simulink model "IIR"  (R2020a)
settings: Solver=ode45  StartTime=0.0  StopTime=10000  RelTol=1e-3  EnableMultiTasking=on
PreLoadFcn:
  | IIR_PreLoadFcn
undefined symbols (not defined in the file): num_channels
libraries: xbsIndex_r4 x125, xbsCopyrightNotice_r4 x1
settings Model: Creator=alexc  LastModifiedBy=viswanad
settings DataIOCC: LimitDataPoints=on  SaveFormat=Array  SignalLoggingSaveFormat=ModelDataLogs  ReturnWorkspaceOutputs=off  SignalLoggingName=sigsOut
settings OptimizationCC: BlockReduction=off  BooleanDataType=off  DefaultParameterBehavior=Inlined  ExpressionDepthLimit=2147483647  InitFltsAndDblsToZero=on  LifeSpan=inf
settings DebuggingCC: SaveWithParameterizedLinksMsg=none  UnderspecifiedInitializationDetection=Classic  MergeDetectMultiDrivingBlocksExec=none  SignalResolutionControl=TryResolveAllWithWarning  MultiTaskDSMMsg=warning  MultiTaskCondExecSysMsg=none  FcnCallInpInsideContextMsg=warning  AllowSymbolicDim=off  StateNameClashWarn=warning  SFUnexpectedBacktrackingDiag=warning  SFNoUnconditionalDefaultTransitionDiag=warning  SFExecutionAtInitializationDiag=none  ArithmeticOperatorsInVariantConditions=warning
settings HardwareCC: ProdBitPerPointer=32  ProdBitPerSizeT=32  ProdBitPerPtrDiffT=32  ProdLargestAtomicFloat=None  ProdIntDivRoundTo=Undefined  ProdEndianess=Unspecified  ProdWordSize=32  ProdHWDeviceType=32-bit Generic  TargetUnknown=on
settings ModelReferenceCC: PropagateSignalLabelsOutOfModel=off
settings SFSimCC: SimUseLocalCustomCode=off  CustomCodeUndefinedFunction=UseInterfaceOnly
settings RTWCC: Description=Generic Real-Time Target  RTWUseLocalCustomCode=off
settings CodeAppCC: StateflowObjectComments=on
settings GRTTargetCC: TargetFcnLib=ansi_tfl_tmw.mat  TargetLangStandard=C89/C90 (ANSI)  CombineOutputUpdateFcns=off  GRTInterface=on
settings ConfigComp: CovMetricSettings=dw  CovSaveCumulativeToWorkspaceVar=on  CovSaveSingleToWorkspaceVar=on  CovExternalEMLEnable=off

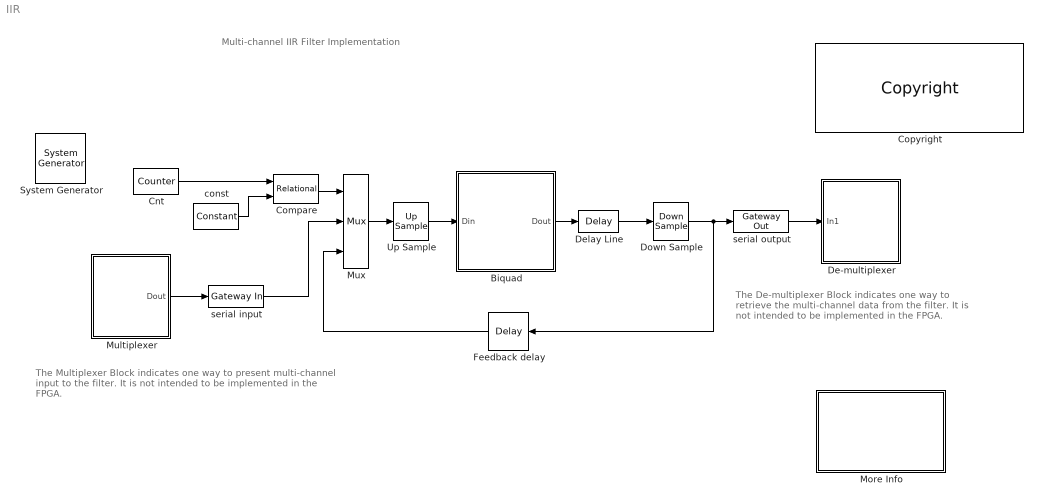
== system IIR ==
  note: Multi-channel IIR Filter Implementation
  note: The Multiplexer Block indicates one way to present
      | multi-channel input to the filter.  It is not intended to
      | be implemented in the FPGA.
  note: The De-multiplexer Block indicates one
      | way to retrieve the multi-channel data
      | from the filter. It is not intended to be
      | implemented in the FPGA.
  " System Generator" : xbsIndex_r4/ System Generator  Tag=genX  xilinxfamily=kintex7  part=xc7k325t  speed=-3  package=fbg676  synthesis_tool=Vivado  clock_wrapper=Clock Enables  directory=./netlist  proj_type=Vivado  Synth_file=Vivado Synthesis Defaults  Impl_file=Vivado Implementation Defaults  testbench=off  simulink_period=1  sysclk_period=22  dcm_input_clock_period=10  incr_netlist=off  trim_vbits=Everywhere in SubSystem  dbl_ovrd=According to Block Masks  core_generation=According to Block Masks  run_coregen=off  deprecated_control=off  eval_field=0  block_type=sysgen
  Biquad : Subsystem
  Cnt : xbsIndex_r4/Counter  cnt_type=Count Limited  cnt_to=4*num_channels-1  operation=Up  start_count=0  cnt_by_val=1  arith_type=Unsigned  n_bits=ceil(log2(4*num_channels))  bin_pt=0  load_pin=off  rst=off  en=off  explicit_period=on  period=5  use_behavioral_HDL=off  implementation=Fabric  use_rpm=off  XmcBlockStatus=1  maskContainerNames=group1  block_type=counter  block_config=sysgen:Counter_config
  Compare : xbsIndex_r4/Relational  mode=a>b  op_type=Bool  en=off  latency=0  XmcBlockStatus=1  maskContainerNames=tabcontainer1  block_type=relational  block_config=sysgen:Relational_config
  Copyright : xbsCopyrightNotice_r4/Copyright  copyrighttext="Copyright (c) 2021  by  Xilinx, Inc. All rights reserved.<br><br>This file contains proprietary, confidential information of Xilinx, Inc., is distributed under license from Xilinx, Inc., and may be used, copied and/or disclosed only pursuant to the terms of a valid license agreement with Xilinx, Inc. Xilinx hereby grants you a license to use this file solely for design, simulation, implementation and creation of design files limited to Xilinx devices or technologies. Use with non-Xilinx devices or technologies is expressly prohibited and immediately terminates your license unless covered by a separate agreement.<br><br>Xilinx is providing this design, code, or information \"as-is\" solely for use in developing programs and solutions for Xilinx devices, with no obligation on the part of Xilinx to provide support. By providing this design, code, or information as one possible implementation of this feature, application or standard, Xilinx is making no representation that this implementation is free from any claims of infringement. You are responsible for obtaining any rights you may require for your implementation. Xilinx expressly disclaims any warranty whatsoever with respect to the adequacy of the implementation, including but not limited to any warranties or representations that this implementation is free from claims of infringement, implied warranties of merchantability or fitness for a particular purpose.<br><br>Xilinx products are not intended for use in life support appliances, devices, or systems. Use in such applications is expressly prohibited.<br><br>Any modifications that are made to the Source Code are done at the user's sole risk and will be unsupported.<br><br>This copyright and support notice must be retained as part of this text at all times. (c) Copyright 1995-2021 Xilinx, Inc. All rights reserved."  block_type=copyright
  De-multiplexer : Subsystem
  Delay Line : xbsIndex_r4/Delay  rst=off  en=off  latency=3  reg_retiming=off  XmcBlockStatus=1  maskContainerNames=group1  block_type=delay  block_config=sysgen:Delay_config
  Down Sample : xbsIndex_r4/Down Sample  sample_ratio=5  sample_phase=First Value of Frame  en=off  rst=off  latency=0  XmcBlockStatus=1  maskContainerNames=group1  block_type=dsamp  block_config=sysgen:Downsample_config
  Feedback delay : xbsIndex_r4/Delay  rst=off  en=off  latency=14  reg_retiming=off  XmcBlockStatus=1  maskContainerNames=group1  block_type=delay  block_config=sysgen:Delay_config
  More Info : Subsystem
      mask Display: disp('Double click\n for\n more information.')
  Multiplexer : Subsystem
  Mux : xbsIndex_r4/Mux  inputs=2  en=off  latency=0  precision=Full  arith_type="Signed  (2's comp)"  n_bits=8  bin_pt=2  quantization=Truncate  overflow=Wrap  XmcBlockStatus=1  maskContainerNames=tabcontainer1  block_type=mux  block_config=sysgen:Mux_config
      settings: infoedit=[]
  Up Sample : xbsIndex_r4/Up Sample  sample_ratio=5  copy_samples=off  en=off  latency=0  XmcBlockStatus=1  maskContainerNames=group1  block_type=usamp  block_config=sysgen:Upsample_config
  const : xbsIndex_r4/Constant  const=num_channels-1  gui_display_data_type=Fixed-point  arith_type=Unsigned  n_bits=ceil(log2(4*num_channels))  bin_pt=0  preci_type=Single  exp_width=8  frac_width=24  explicit_period=off  period=1  XmcBlockStatus=1  maskContainerNames=tabcontainer1  block_type=constant  block_config=sysgen:Constant_config
  serial input : xbsIndex_r4/Gateway In  gui_display_data_type=Fixed-point  arith_type=Signed (2's comp)  n_bits=data_width_nbits  bin_pt=data_width_frac  preci_type=Single  exp_width=8  frac_width=24  rows=1  columns=1  quantization="Round  (unbiased: +/- Inf)"  overflow=Saturate  period=5  UseAsADC=off  ADCChannel='1'  interface=None  automatic_assignment=on  address_offset=hex2dec('00')  intf_name=''  intf_description=''  default_value=0  timing_constraint=Data Rate  locs_specified=off  LOCs={}  io_standard={}  inherit_from_input=off  hdl_port=on  XmcBlockStatus=1  maskContainerNames=group4  block_type=gatewayin  block_config=sysgen:gateway_in_config
  serial output : xbsIndex_r4/Gateway Out  inherit_from_input=off  hdl_port=on  rows=1  columns=1  UseAsDAC=off  DACChannel='1'  interface=None  automatic_assignment=on  address_offset=hex2dec('00')  intf_name=''  intf_description=''  timing_constraint=Data Rate  locs_specified=off  LOCs={}  io_standard={}  XmcBlockStatus=1  maskContainerNames=group4  block_type=gatewayout  block_config=sysgen:gateway_out_config
  wires:
  Biquad/1(Dout) -> Delay Line/1
  Mux/1 -> Up Sample/1
  Feedback delay/1 -> Mux/3
  Up Sample/1 -> Biquad/1(Din)
  Down Sample/1 -> Feedback delay/1, serial output/1
  serial output/1 -> De-multiplexer/1(In1)
  serial input/1 -> Mux/2
  Compare/1 -> Mux/1
  Cnt/1 -> Compare/1
  const/1 -> Compare/2
  Multiplexer/1(Dout) -> serial input/1
  Delay Line/1 -> Down Sample/1

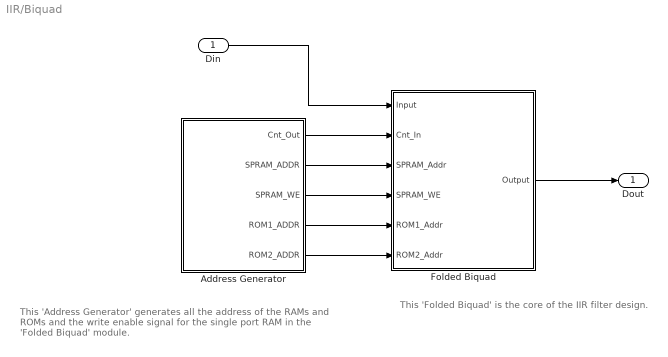
== system IIR/Biquad ==
  note: This 'Address Generator' generates all the address of the
      | RAMs and ROMs and the write enable signal for the single
      | port RAM in the 'Folded Biquad' module.
  note: This 'Folded Biquad' is the core of the IIR filter design.
  Din : Inport
  Address Generator : Subsystem
  Folded Biquad : Subsystem
  Dout : Outport  VectorParamsAs1DForOutWhenUnconnected=off
  wires:
  Address Generator/1(Cnt_Out) -> Folded Biquad/2(Cnt_In)
  Address Generator/2(SPRAM_ADDR) -> Folded Biquad/3(SPRAM_Addr)
  Address Generator/3(SPRAM_WE) -> Folded Biquad/4(SPRAM_WE)
  Address Generator/4(ROM1_ADDR) -> Folded Biquad/5(ROM1_Addr)
  Address Generator/5(ROM2_ADDR) -> Folded Biquad/6(ROM2_Addr)
  Folded Biquad/1(Output) -> Dout/1
  Din/1 -> Folded Biquad/1(Input)

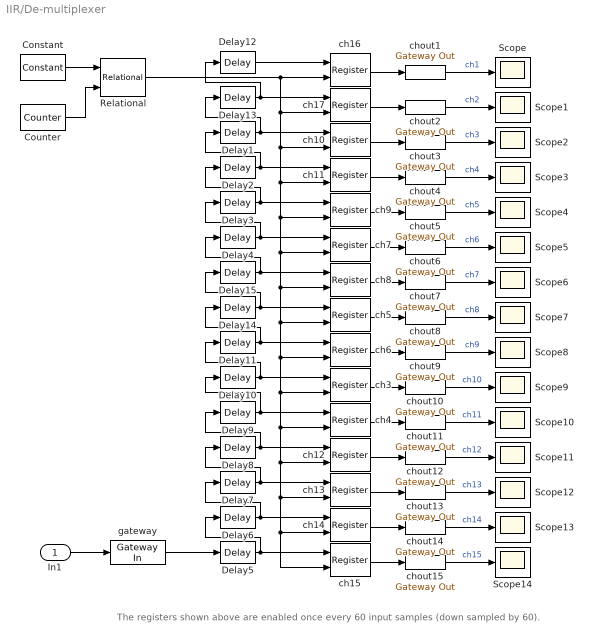
== system IIR/De-multiplexer ==
  note: The registers shown above are enabled once every 60 input samples (down sampled by 60).
  In1 : Inport
  Constant : xbsIndex_r4/Constant  const=0  gui_display_data_type=Fixed-point  arith_type=Unsigned  n_bits=1  bin_pt=0  preci_type=Single  exp_width=8  frac_width=24  explicit_period=off  period=1  XmcBlockStatus=1  maskContainerNames=tabcontainer1  block_type=constant  block_config=sysgen:Constant_config
  Counter : xbsIndex_r4/Counter  cnt_type=Count Limited  cnt_to=4*num_channels-1  operation=Up  start_count=0  cnt_by_val=1  arith_type=Unsigned  n_bits=ceil(log2(4*num_channels))  bin_pt=0  load_pin=off  rst=off  en=off  explicit_period=on  period=5  use_behavioral_HDL=off  implementation=Fabric  use_rpm=off  XmcBlockStatus=1  maskContainerNames=group1  block_type=counter  block_config=sysgen:Counter_config
  Delay{1..15} (15 alike) : xbsIndex_r4/Delay  rst=off  en=off  latency=1  reg_retiming=off  XmcBlockStatus=1  maskContainerNames=group1  block_type=delay  block_config=sysgen:Delay_config
  Relational : xbsIndex_r4/Relational  mode=a=b  op_type=Bool  en=off  latency=0  XmcBlockStatus=1  maskContainerNames=tabcontainer1  block_type=relational  block_config=sysgen:Relational_config
  Scope{,1..14} (15 alike) : Scope
  ch{3..17} (15 alike) : xbsIndex_r4/Register  init=0  rst=off  en=on  XmcBlockStatus=1  maskContainerNames=tabcontainer1  block_type=register  block_config=sysgen:Register_config
  chout{1..15} (15 alike) : xbsIndex_r4/Gateway Out  inherit_from_input=off  hdl_port=off  rows=1  columns=1  UseAsDAC=off  DACChannel='1'  interface=None  automatic_assignment=on  address_offset=hex2dec('00')  intf_name=''  intf_description=''  timing_constraint=Data Rate  locs_specified=off  LOCs={}  io_standard={}  XmcBlockStatus=1  maskContainerNames=group4  block_type=gatewayout  block_config=sysgen:gateway_out_config
  gateway : xbsIndex_r4/Gateway In  gui_display_data_type=Fixed-point  arith_type=Signed (2's comp)  n_bits=data_width_nbits  bin_pt=data_width_frac  preci_type=Single  exp_width=8  frac_width=24  rows=1  columns=1  quantization="Round  (unbiased: +/- Inf)"  overflow=Saturate  period=5  UseAsADC=off  ADCChannel='1'  interface=None  automatic_assignment=on  address_offset=hex2dec('00')  intf_name=''  intf_description=''  default_value=0  timing_constraint=Data Rate  locs_specified=off  LOCs={}  io_standard={}  inherit_from_input=off  hdl_port=on  XmcBlockStatus=1  maskContainerNames=group4  block_type=gatewayin  block_config=sysgen:gateway_in_config
  wires:
  Counter/1 -> Relational/2
  Constant/1 -> Relational/1
  gateway/1 -> Delay5/1
  Delay4/1 -> ch7/1, Delay3/1
  Delay3/1 -> ch9/1, Delay2/1
  Delay2/1 -> ch11/1, Delay1/1
  Delay1/1 -> ch10/1, Delay13/1
  Delay13/1 -> ch17/1, Delay12/1
  Delay12/1 -> ch16/1
  ch16/1 -> chout1/1
  chout1/1 -> Scope/1  "ch1"
  ch17/1 -> chout2/1
  chout2/1 -> Scope1/1  "ch2"
  ch10/1 -> chout3/1
  chout3/1 -> Scope2/1  "ch3"
  ch11/1 -> chout4/1
  chout4/1 -> Scope3/1  "ch4"
  ch9/1 -> chout5/1
  chout5/1 -> Scope4/1  "ch5"
  ch7/1 -> chout6/1
  chout6/1 -> Scope5/1  "ch6"
  chout7/1 -> Scope6/1  "ch7"
  ch8/1 -> chout7/1
  chout8/1 -> Scope7/1  "ch8"
  ch5/1 -> chout8/1
  chout9/1 -> Scope8/1  "ch9"
  ch6/1 -> chout9/1
  chout10/1 -> Scope9/1  "ch10"
  ch3/1 -> chout10/1
  chout11/1 -> Scope10/1  "ch11"
  ch4/1 -> chout11/1
  chout12/1 -> Scope11/1  "ch12"
  ch12/1 -> chout12/1
  chout13/1 -> Scope12/1  "ch13"
  ch13/1 -> chout13/1
  chout14/1 -> Scope13/1  "ch14"
  ch14/1 -> chout14/1
  chout15/1 -> Scope14/1  "ch15"
  ch15/1 -> chout15/1
  In1/1 -> gateway/1
  Relational/1 -> ch15/2, ch14/2, ch13/2, ch12/2, ch4/2, ch3/2, ch6/2, ch5/2, ch8/2, ch7/2, ch9/2, ch11/2, ch10/2, ch17/2, ch16/2
  Delay5/1 -> ch15/1, Delay6/1
  Delay6/1 -> ch14/1, Delay7/1
  Delay7/1 -> ch13/1, Delay8/1
  Delay8/1 -> ch12/1, Delay9/1
  Delay9/1 -> ch4/1, Delay10/1
  Delay10/1 -> ch3/1, Delay11/1
  Delay11/1 -> ch6/1, Delay14/1
  Delay14/1 -> ch5/1, Delay15/1
  Delay15/1 -> ch8/1, Delay4/1

== system IIR/More Info ==
  note: This design demonstrates how multiple IIR filters can be implemented using a single time-shared second-order section (biquad).  Specifically,
      | 15 distinct IIR filters, each consisting of four cascaded biquads, are realized in a "folded" architecture that uses a single hardware biquad.
      | Hardware folding is a technique to time-multiplex many algorithm operations onto a single functional unit (e.g. adder, multiplier).   For low
      | sample rate applications like audio and control, the required silicon area can be much reduced by time-sharing the hardware resources.
      |
      | In this design, the several individual folding techniques are employed:
      |  - the biquad is time-multiplexed among fifteen channels
      |  - the biquad is time-multiplexed among four cascade stages for each channel
      |  - the biquad is implemented using two multipliers and a single adder instead of the straightforward 5 multipliers and 4 adders (a biquad output
      |    is calculated in every 5 system clock cycles).
  note: Multi-channel IIR Filter Implementation

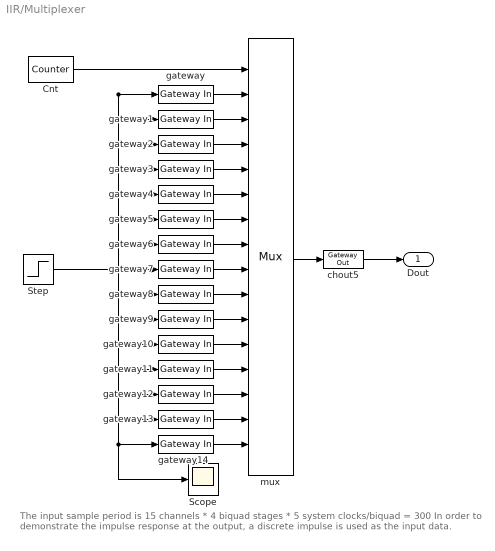
== system IIR/Multiplexer ==
  note: The input sample period is 15 channels * 4 biquad stages * 5 system clocks/biquad = 300
      | In order to demonstrate the impulse response at the output, a discrete impulse is used as
      | the input data.
  Cnt : xbsIndex_r4/Counter  cnt_type=Count Limited  cnt_to=num_channels-1  operation=Up  start_count=0  cnt_by_val=1  arith_type=Unsigned  n_bits=ceil(log2(num_channels))  bin_pt=0  load_pin=off  rst=off  en=off  explicit_period=on  period=5  use_behavioral_HDL=off  implementation=Fabric  use_rpm=off  XmcBlockStatus=1  maskContainerNames=group1  block_type=counter  block_config=sysgen:Counter_config
  Scope : Scope
  Step : Step  Time=300  Before=1  After=0  SampleTime=5
  chout5 : xbsIndex_r4/Gateway Out  inherit_from_input=off  hdl_port=off  rows=1  columns=1  UseAsDAC=off  DACChannel='1'  interface=None  automatic_assignment=on  address_offset=hex2dec('00')  intf_name=''  intf_description=''  timing_constraint=Data Rate  locs_specified=off  LOCs={}  io_standard={}  XmcBlockStatus=1  maskContainerNames=group4  block_type=gatewayout  block_config=sysgen:gateway_out_config
  gateway{,1..14} (15 alike) : xbsIndex_r4/Gateway In  gui_display_data_type=Fixed-point  arith_type=Signed (2's comp)  n_bits=data_width_nbits  bin_pt=data_width_frac  preci_type=Single  exp_width=8  frac_width=24  rows=1  columns=1  quantization="Round  (unbiased: +/- Inf)"  overflow=Saturate  period=5  UseAsADC=off  ADCChannel='1'  interface=None  automatic_assignment=on  address_offset=hex2dec('00')  intf_name=''  intf_description=''  default_value=0  timing_constraint=Data Rate  locs_specified=off  LOCs={}  io_standard={}  inherit_from_input=off  hdl_port=on  XmcBlockStatus=1  maskContainerNames=group4  block_type=gatewayin  block_config=sysgen:gateway_in_config
  mux : xbsIndex_r4/Mux  inputs=15  en=off  latency=0  precision=Full  arith_type="Signed  (2's comp)"  n_bits=8  bin_pt=2  quantization=Truncate  overflow=Wrap  XmcBlockStatus=1  maskContainerNames=tabcontainer1  block_type=mux  block_config=sysgen:Mux_config
      settings: infoedit=[]
  Dout : Outport  VectorParamsAs1DForOutWhenUnconnected=off
  wires:
  mux/1 -> chout5/1
  chout5/1 -> Dout/1
  gateway/1 -> mux/2
  gateway1/1 -> mux/3
  gateway2/1 -> mux/4
  gateway3/1 -> mux/5
  gateway4/1 -> mux/6
  gateway5/1 -> mux/7
  gateway6/1 -> mux/8
  gateway7/1 -> mux/9
  gateway8/1 -> mux/10
  gateway9/1 -> mux/11
  gateway10/1 -> mux/12
  gateway11/1 -> mux/13
  gateway12/1 -> mux/14
  gateway13/1 -> mux/15
  gateway14/1 -> mux/16
  Step/1 -> gateway/1, gateway1/1, gateway3/1, gateway4/1, gateway6/1, gateway7/1, gateway8/1, gateway9/1, gateway10/1, gateway11/1, gateway12/1, gateway13/1, gateway14/1, Scope/1, gateway5/1, gateway2/1
  Cnt/1 -> mux/1

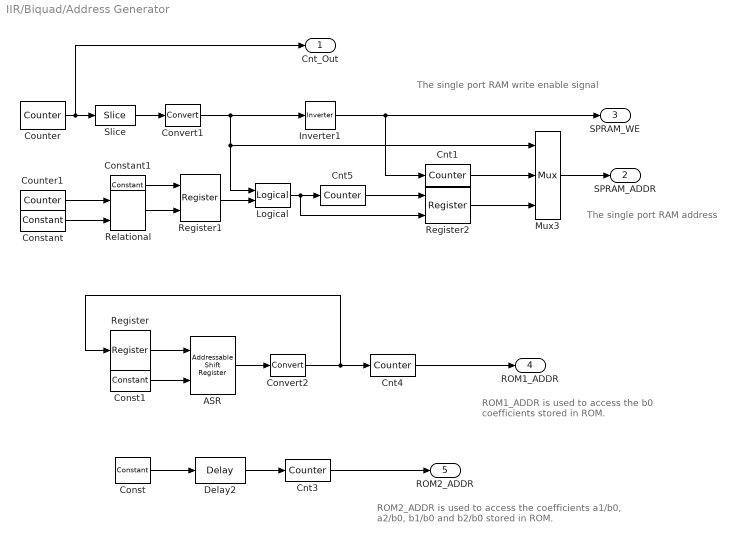
== system IIR/Biquad/Address Generator ==
  note: ROM1_ADDR is used to access
      | the b0 coefficients stored in ROM.
  note: ROM2_ADDR is used to access  the coefficients
      | a1/b0, a2/b0, b1/b0 and b2/b0 stored in ROM.
  note: The single port RAM address
  note: The single port RAM write enable signal
  ASR : xbsIndex_r4/Addressable Shift Register  infer_latency=on  depth=4  initVector=[0 0 0 0]  en=off  use_behavioral_HDL=off  Optimization=Resource  use_rpm=off  XmcBlockStatus=1  maskContainerNames=group1  block_type=addrsr  block_config=sysgen:Addrsr_config
  Cnt1 : xbsIndex_r4/Counter  cnt_type=Count Limited  cnt_to=16*num_channels-1  operation=Up  start_count=0  cnt_by_val=1  arith_type=Unsigned  n_bits=bits_needed_3  bin_pt=0  load_pin=off  rst=off  en=on  explicit_period=off  period=1  use_behavioral_HDL=off  implementation=Fabric  use_rpm=off  XmcBlockStatus=1  maskContainerNames=group1  block_type=counter  block_config=sysgen:Counter_config
  Cnt3 : xbsIndex_r4/Counter  cnt_type=Count Limited  cnt_to=20*num_channels-1  operation=Up  start_count=0  cnt_by_val=1  arith_type=Unsigned  n_bits=bits_needed_2  bin_pt=0  load_pin=off  rst=off  en=on  explicit_period=on  period=1  use_behavioral_HDL=off  implementation=Fabric  use_rpm=off  XmcBlockStatus=1  maskContainerNames=group1  block_type=counter  block_config=sysgen:Counter_config
  Cnt4 : xbsIndex_r4/Counter  cnt_type=Count Limited  cnt_to=4*num_channels-1  operation=Up  start_count=0  cnt_by_val=1  arith_type=Unsigned  n_bits=bits_needed_1  bin_pt=0  load_pin=off  rst=off  en=on  explicit_period=on  period=1  use_behavioral_HDL=off  implementation=Fabric  use_rpm=off  XmcBlockStatus=1  maskContainerNames=group1  block_type=counter  block_config=sysgen:Counter_config
  Cnt5 : xbsIndex_r4/Counter  cnt_type=Count Limited  cnt_to=16*num_channels-1  operation=Up  start_count=3  cnt_by_val=4  arith_type=Unsigned  n_bits=bits_needed_3  bin_pt=0  load_pin=off  rst=off  en=on  explicit_period=off  period=1  use_behavioral_HDL=off  implementation=Fabric  use_rpm=off  XmcBlockStatus=1  maskContainerNames=group1  block_type=counter  block_config=sysgen:Counter_config
  Const : xbsIndex_r4/Constant  const=1  gui_display_data_type=Boolean  arith_type=Boolean  n_bits=1  bin_pt=0  preci_type=Single  exp_width=8  frac_width=24  explicit_period=on  period=1  XmcBlockStatus=1  maskContainerNames=tabcontainer1  block_type=constant  block_config=sysgen:Constant_config
  Const1 : xbsIndex_r4/Constant  const=3  gui_display_data_type=Fixed-point  arith_type=Unsigned  n_bits=2  bin_pt=0  preci_type=Single  exp_width=8  frac_width=24  explicit_period=on  period=1  XmcBlockStatus=1  maskContainerNames=tabcontainer1  block_type=constant  block_config=sysgen:Constant_config
  Constant : xbsIndex_r4/Constant  const=20*num_channels-7  gui_display_data_type=Fixed-point  arith_type=Unsigned  n_bits=9  bin_pt=0  preci_type=Single  exp_width=8  frac_width=24  explicit_period=off  period=1  XmcBlockStatus=1  maskContainerNames=tabcontainer1  block_type=constant  block_config=sysgen:Constant_config
  Constant1 : xbsIndex_r4/Constant  const=1  gui_display_data_type=Boolean  arith_type=Boolean  n_bits=9  bin_pt=0  preci_type=Single  exp_width=8  frac_width=24  explicit_period=off  period=1  XmcBlockStatus=1  maskContainerNames=tabcontainer1  block_type=constant  block_config=sysgen:Constant_config
  Convert1 : xbsIndex_r4/Convert  gui_display_data_type=Boolean  arith_type=Boolean  n_bits=8  bin_pt=6  float_type=Single  exp_bits=8  fraction_bits=24  quantization=Truncate  overflow=Wrap  en=off  latency=0  pipeline=off  XmcBlockStatus=1  maskContainerNames=group2  block_type=convert  block_config=sysgen:Convert_config
  Convert2 : xbsIndex_r4/Convert  gui_display_data_type=Boolean  arith_type=Boolean  n_bits=8  bin_pt=6  float_type=Single  exp_bits=8  fraction_bits=24  quantization=Truncate  overflow=Wrap  en=off  latency=0  pipeline=off  XmcBlockStatus=1  maskContainerNames=group2  block_type=convert  block_config=sysgen:Convert_config
  Counter : xbsIndex_r4/Counter  cnt_type=Count Limited  cnt_to=4  operation=Up  start_count=0  cnt_by_val=1  arith_type=Unsigned  n_bits=3  bin_pt=0  load_pin=off  rst=off  en=off  explicit_period=on  period=1  use_behavioral_HDL=off  implementation=Fabric  use_rpm=off  XmcBlockStatus=1  maskContainerNames=group1  block_type=counter  block_config=sysgen:Counter_config
  Counter1 : xbsIndex_r4/Counter  cnt_type=Free Running  cnt_to=4  operation=Up  start_count=0  cnt_by_val=1  arith_type=Unsigned  n_bits=9  bin_pt=0  load_pin=off  rst=off  en=off  explicit_period=on  period=1  use_behavioral_HDL=off  implementation=Fabric  use_rpm=off  XmcBlockStatus=1  maskContainerNames=group1  block_type=counter  block_config=sysgen:Counter_config
  Delay2 : xbsIndex_r4/Delay  rst=off  en=off  latency=20*num_channels-1  reg_retiming=off  XmcBlockStatus=1  maskContainerNames=group1  block_type=delay  block_config=sysgen:Delay_config
  Inverter1 : xbsIndex_r4/Inverter  en=off  latency=0  XmcBlockStatus=1  maskContainerNames=group2  block_type=inv  block_config=sysgen:Inverter_config
  Logical : xbsIndex_r4/Logical  logical_function=AND  inputs=2  en=off  latency=0  precision=Full  arith_type=Unsigned  n_bits=8  bin_pt=2  align_bp=on  overflow=[]  quantization=[]  XmcBlockStatus=1  maskContainerNames=tabcontainer1  block_type=logical  block_config=sysgen:Logical_config
  Mux3 : xbsIndex_r4/Mux  inputs=2  en=off  latency=0  precision=User Defined  arith_type=Unsigned  n_bits=bits_needed_3  bin_pt=0  quantization=Truncate  overflow=Flag as error  XmcBlockStatus=1  maskContainerNames=tabcontainer1  block_type=mux  block_config=sysgen:Mux_config
      settings: infoedit=[]
  Register : xbsIndex_r4/Register  init=1  rst=off  en=off  XmcBlockStatus=1  maskContainerNames=tabcontainer1  block_type=register  block_config=sysgen:Register_config
  Register1 : xbsIndex_r4/Register  init=0  rst=off  en=on  XmcBlockStatus=1  maskContainerNames=tabcontainer1  block_type=register  block_config=sysgen:Register_config
  Register2 : xbsIndex_r4/Register  init=0  rst=off  en=on  XmcBlockStatus=1  maskContainerNames=tabcontainer1  block_type=register  block_config=sysgen:Register_config
  Relational : xbsIndex_r4/Relational  mode=a=b  op_type=Bool  en=off  latency=0  XmcBlockStatus=1  maskContainerNames=tabcontainer1  block_type=relational  block_config=sysgen:Relational_config
  Slice : xbsIndex_r4/Slice  nbits=1  boolean_output=off  mode=Upper Bit Location + Width  bit1=0  base1=MSB of Input  bit0=0  base0=LSB of Input  XmcBlockStatus=1  maskContainerNames=group1  block_type=slice  block_config=sysgen:Slice_config
  Cnt_Out : Outport  VectorParamsAs1DForOutWhenUnconnected=off
  SPRAM_ADDR : Outport  Port=2  VectorParamsAs1DForOutWhenUnconnected=off
  SPRAM_WE : Outport  Port=3  VectorParamsAs1DForOutWhenUnconnected=off
  ROM1_ADDR : Outport  Port=4  VectorParamsAs1DForOutWhenUnconnected=off
  ROM2_ADDR : Outport  Port=5  VectorParamsAs1DForOutWhenUnconnected=off
  wires:
  Delay2/1 -> Cnt3/1
  Cnt3/1 -> ROM2_ADDR/1
  Const/1 -> Delay2/1
  Convert2/1 -> Register/1, Cnt4/1
  ASR/1 -> Convert2/1
  Register/1 -> ASR/1
  Const1/1 -> ASR/2
  Cnt4/1 -> ROM1_ADDR/1
  Inverter1/1 -> SPRAM_WE/1, Cnt1/1
  Convert1/1 -> Mux3/1, Logical/1, Inverter1/1
  Slice/1 -> Convert1/1
  Counter/1 -> Cnt_Out/1, Slice/1
  Mux3/1 -> SPRAM_ADDR/1
  Cnt1/1 -> Mux3/2
  Counter1/1 -> Relational/1
  Constant/1 -> Relational/2
  Relational/1 -> Register1/2
  Constant1/1 -> Register1/1
  Register1/1 -> Logical/2
  Logical/1 -> Cnt5/1, Register2/2
  Cnt5/1 -> Register2/1
  Register2/1 -> Mux3/3

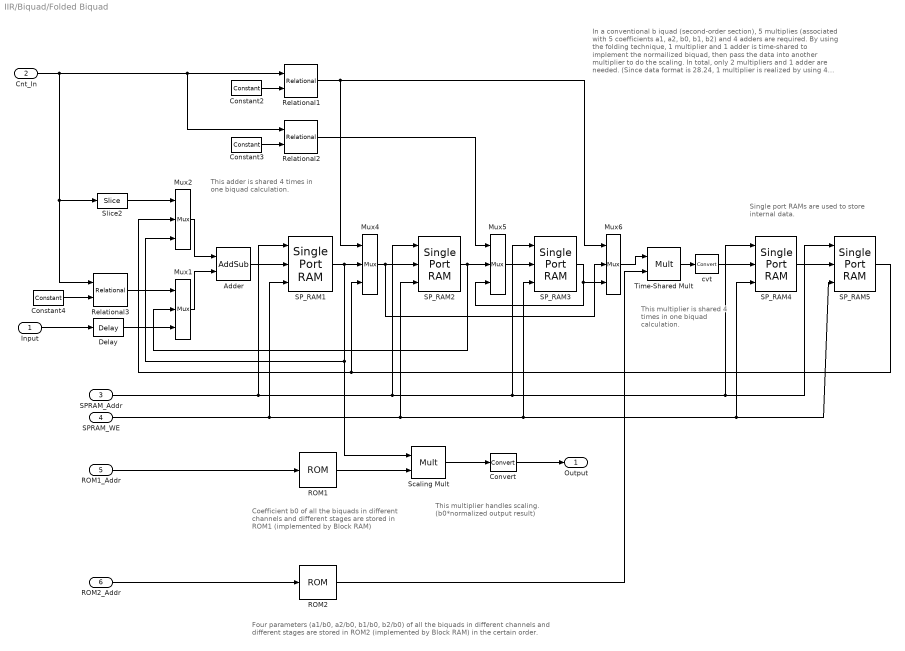
== system IIR/Biquad/Folded Biquad ==
  note: Coefficient b0 of all the biquads in
      | different channels and different stages
      | are stored in ROM1 (implemented by
      | Block RAM)
  note: Four parameters (a1/b0, a2/b0, b1/b0, b2/b0) of all the biquads in different
      | channels and different stages are stored in ROM2 (implemented by Block RAM)
      | in the certain order.
  note: In a conventional b   iquad (second-order section), 5 multiplies
      | (associated with 5 coefficients a1, a2, b0, b1, b2) and 4 adders
      | are required.  By using the folding technique, 1 multiplier and
      | 1 adder is time-shared to implement the normailized biquad,
      | then pass the data into another multiplier to do the scaling.
      | In total, only 2 multipliers and 1 adder are needed. (Since
      | data format is 28.24, 1 multiplier is realized by using
      | 4 18x18 embedded multipliers )
  note: This multiplier is
      | shared 4 times in
      | one biquad
      | calculation.
  note: This adder is
      | shared 4 times
      | in one biquad
      | calculation.
  note: Single port RAMs are used to store
      | internal data.
  note: This multiplier handles scaling.
      | (b0*normalized output result)
  Input : Inport
  Cnt_In : Inport  Port=2
  SPRAM_Addr : Inport  Port=3
  SPRAM_WE : Inport  Port=4
  ROM1_Addr : Inport  Port=5
  ROM2_Addr : Inport  Port=6
  Adder : xbsIndex_r4/AddSub  mode=Addition  use_carryin=off  use_carryout=off  en=off  latency=0  precision=User Defined  arith_type="Signed  (2's comp)"  n_bits=data_width_nbits  bin_pt=data_width_frac  quantization="Round  (unbiased: +/- Inf)"  overflow=Flag as error  use_behavioral_HDL=on  hw_selection=Fabric  pipelined=off  use_rpm=off  XmcBlockStatus=1  maskContainerNames=tabcontainer1  block_type=addsub  block_config=sysgen:Addsub_config
  Constant2 : xbsIndex_r4/Constant  const=0  gui_display_data_type=Fixed-point  arith_type=Unsigned  n_bits=1  bin_pt=0  preci_type=Single  exp_width=8  frac_width=24  explicit_period=off  period=1  XmcBlockStatus=1  maskContainerNames=tabcontainer1  block_type=constant  block_config=sysgen:Constant_config
  Constant3 : xbsIndex_r4/Constant  const=1  gui_display_data_type=Fixed-point  arith_type=Unsigned  n_bits=1  bin_pt=0  preci_type=Single  exp_width=8  frac_width=24  explicit_period=off  period=1  XmcBlockStatus=1  maskContainerNames=tabcontainer1  block_type=constant  block_config=sysgen:Constant_config
  Constant4 : xbsIndex_r4/Constant  const=3  gui_display_data_type=Fixed-point  arith_type=Unsigned  n_bits=2  bin_pt=0  preci_type=Single  exp_width=8  frac_width=24  explicit_period=off  period=1  XmcBlockStatus=1  maskContainerNames=tabcontainer1  block_type=constant  block_config=sysgen:Constant_config
  Convert : xbsIndex_r4/Convert  gui_display_data_type=Fixed-point  arith_type=Signed (2's comp)  n_bits=data_width_nbits  bin_pt=data_width_frac  float_type=Single  exp_bits=8  fraction_bits=24  quantization=Truncate  overflow=Wrap  en=off  latency=0  pipeline=off  XmcBlockStatus=1  maskContainerNames=group2  block_type=convert  block_config=sysgen:Convert_config
  Delay : xbsIndex_r4/Delay  rst=off  en=off  latency=3  reg_retiming=off  XmcBlockStatus=1  maskContainerNames=group1  block_type=delay  block_config=sysgen:Delay_config
  Mux{1..2,4..6} (5 alike) : xbsIndex_r4/Mux  inputs=2  en=off  latency=0  precision=User Defined  arith_type="Signed  (2's comp)"  n_bits=data_width_nbits  bin_pt=data_width_frac  quantization=Truncate  overflow=Flag as error  XmcBlockStatus=1  maskContainerNames=tabcontainer1  block_type=mux  block_config=sysgen:Mux_config
      settings: infoedit=[]
  ROM1 : xbsIndex_r4/ROM  depth=4*num_channels  initVector=coeff_b0  distributed_mem=Block RAM  rst=off  init_reg=0  en=off  latency=2  optimize_latency=off  gui_display_data_type=Fixed-point  arith_type="Signed  (2's comp)"  n_bits=data_width_nbits  bin_pt=data_width_frac  preci_type=Single  exp_width=8  frac_width=24  optimize=Area  use_rpm=off  simulation_type=fast_sim  XmcBlockStatus=1  maskContainerNames=tabcontainer1  block_type=sprom  block_config=sysgen:SPROM_config
  ROM2 : xbsIndex_r4/ROM  depth=20*num_channels  initVector=coeffs  distributed_mem=Block RAM  rst=off  init_reg=0  en=off  latency=1  optimize_latency=off  gui_display_data_type=Fixed-point  arith_type="Signed  (2's comp)"  n_bits=data_width_nbits  bin_pt=data_width_frac  preci_type=Single  exp_width=8  frac_width=24  optimize=Area  use_rpm=off  simulation_type=fast_sim  XmcBlockStatus=1  maskContainerNames=tabcontainer1  block_type=sprom  block_config=sysgen:SPROM_config
  Relational1 : xbsIndex_r4/Relational  mode=a!=b  op_type=Bool  en=off  latency=0  XmcBlockStatus=1  maskContainerNames=tabcontainer1  block_type=relational  block_config=sysgen:Relational_config
  Relational2 : xbsIndex_r4/Relational  mode=a!=b  op_type=Bool  en=off  latency=0  XmcBlockStatus=1  maskContainerNames=tabcontainer1  block_type=relational  block_config=sysgen:Relational_config
  Relational3 : xbsIndex_r4/Relational  mode=a=b  op_type=Bool  en=off  latency=0  XmcBlockStatus=1  maskContainerNames=tabcontainer1  block_type=relational  block_config=sysgen:Relational_config
  SP_RAM{1..5} (5 alike) : xbsIndex_r4/Single Port RAM  depth=16*num_channels  initVector=[zeros([1,16*num_channels])]  distributed_mem=Block RAM  write_mode=Read After Write  rst=off  init_reg=0  en=off  optimize_latency=off  latency=1  optimize=Area  dbl_ovrd=off  simulation_type=fast_sim  XmcBlockStatus=1  maskContainerNames=tabcontainer1  block_type=spram  block_config=sysgen:SPRAM_config
      SP_RAM2 settings: xl_area=[0 0 1 0 0 0 0]
      SP_RAM3 settings: xl_area=[0 0 1 0 0 0 0]
      SP_RAM4 settings: xl_area=[0 0 1 0 0 0 0]
      SP_RAM5 settings: xl_area=[0 0 1 0 0 0 0]
  Scaling Mult : xbsIndex_r4/Mult  precision=User Defined  arith_type="Signed  (2's comp)"  n_bits=mult_width_nbits  bin_pt=mult_width_frac  quantization=Truncate  overflow=Flag as error  en=off  latency=0  use_behavioral_HDL=off  opt=Speed  use_embedded=on  optimum_pipeline=off  pipeline=off  use_rpm=off  placement_style=Rectangular shape  XmcBlockStatus=1  maskContainerNames=group1  block_type=mult  block_config=sysgen:Mult_config
  Slice2 : xbsIndex_r4/Slice  nbits=1  boolean_output=off  mode=Lower Bit Location + Width  bit1=0  base1=MSB of Input  bit0=0  base0=LSB of Input  XmcBlockStatus=1  maskContainerNames=group1  block_type=slice  block_config=sysgen:Slice_config
  Time-Shared Mult : xbsIndex_r4/Mult  precision=Full  arith_type="Signed  (2's comp)"  n_bits=mult_width_nbits  bin_pt=mult_width_frac  quantization=Truncate  overflow=Flag as error  en=off  latency=0  use_behavioral_HDL=off  opt=Speed  use_embedded=on  optimum_pipeline=off  pipeline=off  use_rpm=off  placement_style=Rectangular shape  XmcBlockStatus=1  maskContainerNames=group1  block_type=mult  block_config=sysgen:Mult_config
  cvt : xbsIndex_r4/Convert  gui_display_data_type=Fixed-point  arith_type=Signed (2's comp)  n_bits=data_width_nbits  bin_pt=data_width_frac  float_type=Single  exp_bits=8  fraction_bits=24  quantization=Truncate  overflow=Wrap  en=off  latency=0  pipeline=off  XmcBlockStatus=1  maskContainerNames=group2  block_type=convert  block_config=sysgen:Convert_config
  Output : Outport  VectorParamsAs1DForOutWhenUnconnected=off
  wires:
  Time-Shared Mult/1 -> cvt/1
  Adder/1 -> SP_RAM1/2
  SP_RAM2/1 -> Mux5/2, Mux1/2
  Input/1 -> Delay/1
  Mux4/1 -> Mux6/2, SP_RAM2/2
  Mux5/1 -> SP_RAM3/2
  SP_RAM3/1 -> Mux6/3, Mux5/3
  cvt/1 -> SP_RAM4/2
  Delay/1 -> Mux1/3
  SP_RAM4/1 -> SP_RAM5/2
  Cnt_In/1 -> Relational1/1, Relational2/1, Relational3/1, Slice2/1
  SP_RAM1/1 -> Mux4/2, Mux2/3, Scaling Mult/1
  Constant2/1 -> Relational1/2
  Constant3/1 -> Relational2/2
  Relational2/1 -> Mux5/1
  Mux2/1 -> Adder/1
  Mux1/1 -> Adder/2
  Constant4/1 -> Relational3/2
  Relational3/1 -> Mux1/1
  Mux6/1 -> Time-Shared Mult/1
  SP_RAM5/1 -> Mux2/2, Mux4/3
  Slice2/1 -> Mux2/1
  ROM2/1 -> Time-Shared Mult/2
  Relational1/1 -> Mux4/1, Mux6/1
  Scaling Mult/1 -> Convert/1
  Convert/1 -> Output/1
  ROM1/1 -> Scaling Mult/2
  SPRAM_Addr/1 -> SP_RAM5/1, SP_RAM4/1, SP_RAM3/1, SP_RAM2/1, SP_RAM1/1
  SPRAM_WE/1 -> SP_RAM2/3, SP_RAM5/3, SP_RAM4/3, SP_RAM3/3, SP_RAM1/3
  ROM2_Addr/1 -> ROM2/1
  ROM1_Addr/1 -> ROM1/1
